simulink model "proba1"  (R2017b)
settings: Solver=VariableStepAuto  StartTime=0.0  StopTime=120  RelTol=1e-3  EnableMultiTasking=on
libraries: xbsIndex_r4 x61
settings Model: Creator=szekelyi  LastModifiedBy=kovacs.attila
settings DataIOCC: LimitDataPoints=on
settings OptimizationCC: LifeSpan=inf
settings DebuggingCC: AllowSymbolicDim=off  SFUnexpectedBacktrackingDiag=warning  SFNoUnconditionalDefaultTransitionDiag=warning  SFExecutionAtInitializationDiag=none
settings ModelReferenceCC: PropagateSignalLabelsOutOfModel=off
settings CodeAppCC: StateflowObjectComments=on
settings GRTTargetCC: TargetLangStandard=C89/C90 (ANSI)
settings ConfigComp: CovMetricSettings=dw  CovHtmlReporting=on  CovSaveCumulativeToWorkspaceVar=on  CovSaveSingleToWorkspaceVar=on  CovExternalEMLEnable=off

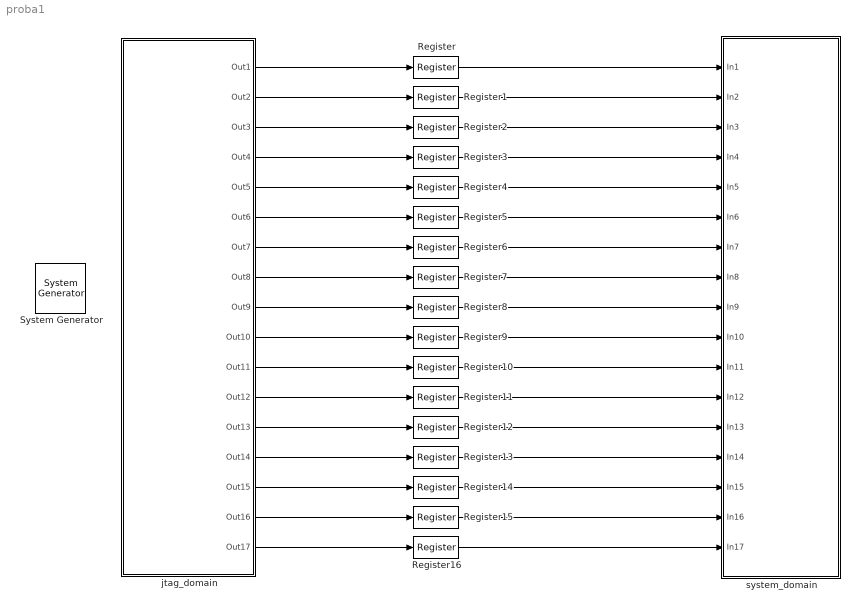
== system proba1 ==
  " System Generator" : xbsIndex_r4/ System Generator  Tag=genX  xilinxfamily=artix7  part=xc7a35t  speed=-1  package=cpg236  synthesis_tool=Vivado  clock_wrapper=Clock Enables  directory=./netlist  proj_type=Vivado  Synth_file=Vivado Synthesis Defaults  Impl_file=Vivado Implementation Defaults  testbench=off  simulink_period=1  sysclk_period=10  dcm_input_clock_period=10  incr_netlist=off  trim_vbits=Everywhere in SubSystem  dbl_ovrd=According to Block Masks  core_generation=According to Block Masks  run_coregen=off  deprecated_control=off  eval_field=0  block_type=sysgen
  Register{,1..16} (17 alike) : xbsIndex_r4/Register  init=0  rst=off  en=off  dbl_ovrd=off  block_type=register
  jtag_domain : Subsystem
  system_domain : Subsystem
  wires:
  jtag_domain/1(Out1) -> Register/1
  jtag_domain/2(Out2) -> Register1/1
  jtag_domain/3(Out3) -> Register2/1
  jtag_domain/4(Out4) -> Register3/1
  jtag_domain/5(Out5) -> Register4/1
  jtag_domain/6(Out6) -> Register5/1
  Register/1 -> system_domain/1(In1)
  Register1/1 -> system_domain/2(In2)
  Register2/1 -> system_domain/3(In3)
  Register3/1 -> system_domain/4(In4)
  Register4/1 -> system_domain/5(In5)
  Register5/1 -> system_domain/6(In6)
  Register11/1 -> system_domain/12(In12)
  Register9/1 -> system_domain/10(In10)
  jtag_domain/11(Out11) -> Register10/1
  Register10/1 -> system_domain/11(In11)
  Register8/1 -> system_domain/9(In9)
  Register7/1 -> system_domain/8(In8)
  Register6/1 -> system_domain/7(In7)
  jtag_domain/12(Out12) -> Register11/1
  jtag_domain/10(Out10) -> Register9/1
  jtag_domain/8(Out8) -> Register7/1
  jtag_domain/9(Out9) -> Register8/1
  jtag_domain/7(Out7) -> Register6/1
  Register15/1 -> system_domain/16(In16)
  jtag_domain/17(Out17) -> Register16/1
  Register16/1 -> system_domain/17(In17)
  Register14/1 -> system_domain/15(In15)
  Register13/1 -> system_domain/14(In14)
  Register12/1 -> system_domain/13(In13)
  jtag_domain/16(Out16) -> Register15/1
  jtag_domain/14(Out14) -> Register13/1
  jtag_domain/15(Out15) -> Register14/1
  jtag_domain/13(Out13) -> Register12/1

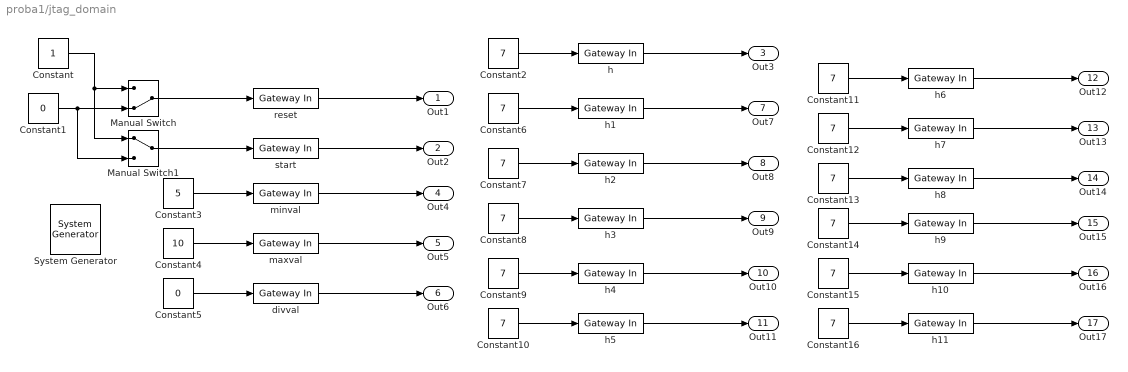
== system proba1/jtag_domain ==
  " System Generator" : xbsIndex_r4/ System Generator  Tag=genX  xilinxfamily=artix7  part=xc7a35t  speed=-1  package=cpg236  synthesis_tool=Vivado  clock_wrapper=Clock Enables  directory=./netlist  proj_type=Vivado  Synth_file=Vivado Synthesis Defaults  Impl_file=Vivado Implementation Defaults  testbench=off  simulink_period=1  sysclk_period=10  dcm_input_clock_period=10  incr_netlist=off  trim_vbits=Everywhere in SubSystem  dbl_ovrd=According to Block Masks  core_generation=According to Block Masks  run_coregen=off  deprecated_control=off  eval_field=0  block_type=sysgen
  Constant : Constant
  Constant1 : Constant  Value=0
  Constant{2,6..16} (12 alike) : Constant  Value=7
  Constant3 : Constant  Value=5
  Constant4 : Constant  Value=10
  Constant5 : Constant  Value=0
  Manual Switch : ManualSwitch  CurrentSetting=0
  Manual Switch1 : ManualSwitch
  divval : xbsIndex_r4/Gateway In  gui_display_data_type=Fixed-point  arith_type=Unsigned  n_bits=10  bin_pt=0  preci_type=Single  exp_width=8  frac_width=24  rows=1  columns=1  quantization="Round  (unbiased: +/- Inf)"  overflow=Saturate  period=1  UseAsADC=off  ADCChannel='1'  interface=None  automatic_assignment=on  address_offset=hex2dec('00')  intf_name=''  intf_description=''  default_value=0  timing_constraint=None  locs_specified=off  LOCs={}  io_standard={}  inherit_from_input=off  hdl_port=on  dbl_ovrd=off  block_type=gatewayin
  h{,1..11} (12 alike) : xbsIndex_r4/Gateway In  gui_display_data_type=Fixed-point  arith_type=Unsigned  n_bits=32  bin_pt=0  preci_type=Single  exp_width=8  frac_width=24  rows=1  columns=1  quantization="Round  (unbiased: +/- Inf)"  overflow=Saturate  period=1  UseAsADC=off  ADCChannel='1'  interface=None  automatic_assignment=on  address_offset=hex2dec('00')  intf_name=''  intf_description=''  default_value=0  timing_constraint=None  locs_specified=off  LOCs={}  io_standard={}  inherit_from_input=off  hdl_port=on  dbl_ovrd=off  block_type=gatewayin
  maxval : xbsIndex_r4/Gateway In  gui_display_data_type=Fixed-point  arith_type=Unsigned  n_bits=32  bin_pt=0  preci_type=Single  exp_width=8  frac_width=24  rows=1  columns=1  quantization="Round  (unbiased: +/- Inf)"  overflow=Saturate  period=1  UseAsADC=off  ADCChannel='1'  interface=None  automatic_assignment=on  address_offset=hex2dec('00')  intf_name=''  intf_description=''  default_value=0  timing_constraint=None  locs_specified=off  LOCs={}  io_standard={}  inherit_from_input=off  hdl_port=on  dbl_ovrd=off  block_type=gatewayin
  minval : xbsIndex_r4/Gateway In  gui_display_data_type=Fixed-point  arith_type=Unsigned  n_bits=32  bin_pt=0  preci_type=Single  exp_width=8  frac_width=24  rows=1  columns=1  quantization="Round  (unbiased: +/- Inf)"  overflow=Saturate  period=1  UseAsADC=off  ADCChannel='1'  interface=None  automatic_assignment=on  address_offset=hex2dec('00')  intf_name=''  intf_description=''  default_value=0  timing_constraint=None  locs_specified=off  LOCs={}  io_standard={}  inherit_from_input=off  hdl_port=on  dbl_ovrd=off  block_type=gatewayin
  reset : xbsIndex_r4/Gateway In  gui_display_data_type=Boolean  arith_type=Boolean  n_bits=16  bin_pt=14  preci_type=Single  exp_width=8  frac_width=24  rows=1  columns=1  quantization="Round  (unbiased: +/- Inf)"  overflow=Saturate  period=1  UseAsADC=off  ADCChannel='1'  interface=None  automatic_assignment=on  address_offset=hex2dec('00')  intf_name=''  intf_description=''  default_value=0  timing_constraint=None  locs_specified=off  LOCs={}  io_standard={}  inherit_from_input=off  hdl_port=on  dbl_ovrd=off  block_type=gatewayin
  start : xbsIndex_r4/Gateway In  gui_display_data_type=Boolean  arith_type=Boolean  n_bits=16  bin_pt=14  preci_type=Single  exp_width=8  frac_width=24  rows=1  columns=1  quantization="Round  (unbiased: +/- Inf)"  overflow=Saturate  period=1  UseAsADC=off  ADCChannel='1'  interface=None  automatic_assignment=on  address_offset=hex2dec('00')  intf_name=''  intf_description=''  default_value=0  timing_constraint=None  locs_specified=off  LOCs={}  io_standard={}  inherit_from_input=off  hdl_port=on  dbl_ovrd=off  block_type=gatewayin
  Out1 : Outport
  Out2 : Outport  Port=2
  Out3 : Outport  Port=3
  Out4 : Outport  Port=4
  Out5 : Outport  Port=5
  Out6 : Outport  Port=6
  Out7 : Outport  Port=7
  Out8 : Outport  Port=8
  Out9 : Outport  Port=9
  Out10 : Outport  Port=10
  Out11 : Outport  Port=11
  Out12 : Outport  Port=12
  Out13 : Outport  Port=13
  Out14 : Outport  Port=14
  Out15 : Outport  Port=15
  Out16 : Outport  Port=16
  Out17 : Outport  Port=17
  wires:
  h/1 -> Out3/1
  start/1 -> Out2/1
  maxval/1 -> Out5/1
  minval/1 -> Out4/1
  divval/1 -> Out6/1
  reset/1 -> Out1/1
  Manual Switch/1 -> reset/1
  Manual Switch1/1 -> start/1
  Constant/1 -> Manual Switch1/1, Manual Switch/1
  Constant1/1 -> Manual Switch1/2, Manual Switch/2
  Constant2/1 -> h/1
  Constant3/1 -> minval/1
  Constant4/1 -> maxval/1
  Constant5/1 -> divval/1
  Constant6/1 -> h1/1
  h1/1 -> Out7/1
  Constant7/1 -> h2/1
  h2/1 -> Out8/1
  Constant8/1 -> h3/1
  h3/1 -> Out9/1
  Constant9/1 -> h4/1
  h4/1 -> Out10/1
  Constant10/1 -> h5/1
  h5/1 -> Out11/1
  Constant11/1 -> h6/1
  h6/1 -> Out12/1
  Constant12/1 -> h7/1
  h7/1 -> Out13/1
  Constant13/1 -> h8/1
  h8/1 -> Out14/1
  Constant14/1 -> h9/1
  h9/1 -> Out15/1
  Constant15/1 -> h10/1
  h10/1 -> Out16/1
  Constant16/1 -> h11/1
  h11/1 -> Out17/1

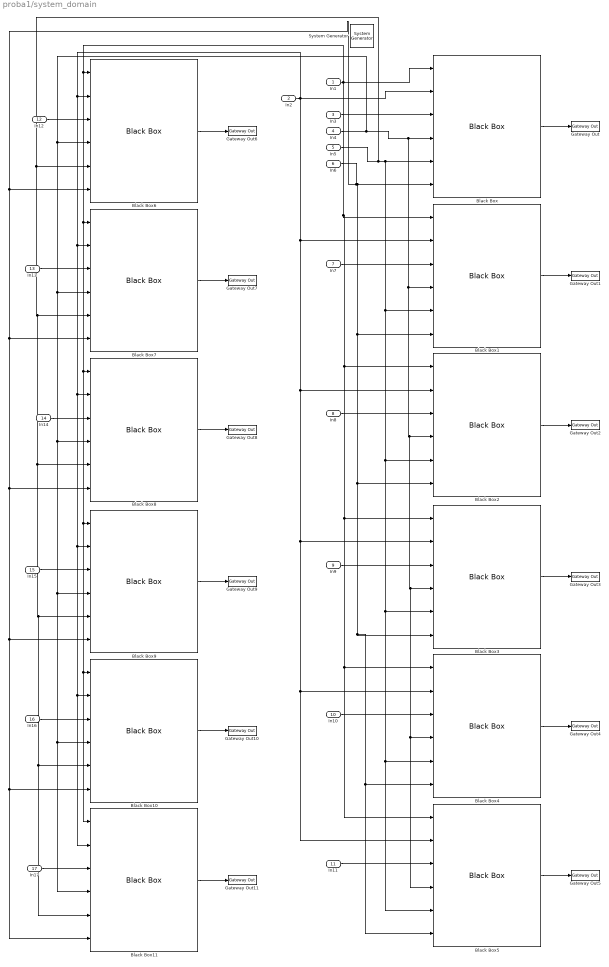
== system proba1/system_domain ==
  In1 : Inport
  In2 : Inport  Port=2
  In3 : Inport  Port=3
  In4 : Inport  Port=4
  In5 : Inport  Port=5
  In6 : Inport  Port=6
  In7 : Inport  Port=7
  In8 : Inport  Port=8
  In9 : Inport  Port=9
  In10 : Inport  Port=10
  In11 : Inport  Port=11
  In12 : Inport  Port=12
  In13 : Inport  Port=13
  In14 : Inport  Port=14
  In15 : Inport  Port=15
  In16 : Inport  Port=16
  In17 : Inport  Port=17
  " System Generator" : xbsIndex_r4/ System Generator  Tag=genX  xilinxfamily=artix7  part=xc7a35t  speed=-1  package=cpg236  synthesis_tool=Vivado  clock_wrapper=Clock Enables  directory=./netlist  proj_type=Vivado  Synth_file=Vivado Synthesis Defaults  Impl_file=Vivado Implementation Defaults  testbench=off  simulink_period=1  sysclk_period=10  dcm_input_clock_period=10  incr_netlist=off  trim_vbits=Everywhere in SubSystem  dbl_ovrd=According to Block Masks  core_generation=According to Block Masks  run_coregen=off  deprecated_control=off  eval_field=0  block_type=sysgen
  Black Box{,1..11} (12 alike) : xbsIndex_r4/Black Box  init_code=pwm_ultra_config  sim_method=ISE Simulator  verbose=off  block_type=blackbox2
  Gateway Out : xbsIndex_r4/Gateway Out  inherit_from_input=off  hdl_port=on  rows=1  columns=1  UseAsDAC=off  DACChannel='1'  interface=None  automatic_assignment=on  address_offset=hex2dec('00')  intf_name=''  intf_description=''  timing_constraint=None  locs_specified=on  LOCs={'M3'}  io_standard={'LVCMOS33'}  block_type=gatewayout
  Gateway Out1 : xbsIndex_r4/Gateway Out  inherit_from_input=off  hdl_port=on  rows=1  columns=1  UseAsDAC=off  DACChannel='1'  interface=None  automatic_assignment=on  address_offset=hex2dec('00')  intf_name=''  intf_description=''  timing_constraint=None  locs_specified=on  LOCs={'L3'}  io_standard={'LVCMOS33'}  block_type=gatewayout
  Gateway Out10 : xbsIndex_r4/Gateway Out  inherit_from_input=off  hdl_port=on  rows=1  columns=1  UseAsDAC=off  DACChannel='1'  interface=None  automatic_assignment=on  address_offset=hex2dec('00')  intf_name=''  intf_description=''  timing_constraint=None  locs_specified=on  LOCs={'J1'}  io_standard={'LVCMOS33'}  block_type=gatewayout
  Gateway Out11 : xbsIndex_r4/Gateway Out  inherit_from_input=off  hdl_port=on  rows=1  columns=1  UseAsDAC=off  DACChannel='1'  interface=None  automatic_assignment=on  address_offset=hex2dec('00')  intf_name=''  intf_description=''  timing_constraint=None  locs_specified=on  LOCs={'K2'}  io_standard={'LVCMOS33'}  block_type=gatewayout
  Gateway Out2 : xbsIndex_r4/Gateway Out  inherit_from_input=off  hdl_port=on  rows=1  columns=1  UseAsDAC=off  DACChannel='1'  interface=None  automatic_assignment=on  address_offset=hex2dec('00')  intf_name=''  intf_description=''  timing_constraint=None  locs_specified=on  LOCs={'A16'}  io_standard={'LVCMOS33'}  block_type=gatewayout
  Gateway Out3 : xbsIndex_r4/Gateway Out  inherit_from_input=off  hdl_port=on  rows=1  columns=1  UseAsDAC=off  DACChannel='1'  interface=None  automatic_assignment=on  address_offset=hex2dec('00')  intf_name=''  intf_description=''  timing_constraint=None  locs_specified=on  LOCs={'K3'}  io_standard={'LVCMOS33'}  block_type=gatewayout
  Gateway Out4 : xbsIndex_r4/Gateway Out  inherit_from_input=off  hdl_port=on  rows=1  columns=1  UseAsDAC=off  DACChannel='1'  interface=None  automatic_assignment=on  address_offset=hex2dec('00')  intf_name=''  intf_description=''  timing_constraint=None  locs_specified=on  LOCs={'C15'}  io_standard={'LVCMOS33'}  block_type=gatewayout
  Gateway Out5 : xbsIndex_r4/Gateway Out  inherit_from_input=off  hdl_port=on  rows=1  columns=1  UseAsDAC=off  DACChannel='1'  interface=None  automatic_assignment=on  address_offset=hex2dec('00')  intf_name=''  intf_description=''  timing_constraint=None  locs_specified=on  LOCs={'H1'}  io_standard={'LVCMOS33'}  block_type=gatewayout
  Gateway Out6 : xbsIndex_r4/Gateway Out  inherit_from_input=off  hdl_port=on  rows=1  columns=1  UseAsDAC=off  DACChannel='1'  interface=None  automatic_assignment=on  address_offset=hex2dec('00')  intf_name=''  intf_description=''  timing_constraint=None  locs_specified=on  LOCs={'A15'}  io_standard={'LVCMOS33'}  block_type=gatewayout
  Gateway Out7 : xbsIndex_r4/Gateway Out  inherit_from_input=off  hdl_port=on  rows=1  columns=1  UseAsDAC=off  DACChannel='1'  interface=None  automatic_assignment=on  address_offset=hex2dec('00')  intf_name=''  intf_description=''  timing_constraint=None  locs_specified=on  LOCs={'B15'}  io_standard={'LVCMOS33'}  block_type=gatewayout
  Gateway Out8 : xbsIndex_r4/Gateway Out  inherit_from_input=off  hdl_port=on  rows=1  columns=1  UseAsDAC=off  DACChannel='1'  interface=None  automatic_assignment=on  address_offset=hex2dec('00')  intf_name=''  intf_description=''  timing_constraint=None  locs_specified=on  LOCs={'A14'}  io_standard={'LVCMOS33'}  block_type=gatewayout
  Gateway Out9 : xbsIndex_r4/Gateway Out  inherit_from_input=off  hdl_port=on  rows=1  columns=1  UseAsDAC=off  DACChannel='1'  interface=None  automatic_assignment=on  address_offset=hex2dec('00')  intf_name=''  intf_description=''  timing_constraint=None  locs_specified=on  LOCs={'J3'}  io_standard={'LVCMOS33'}  block_type=gatewayout
  wires:
  Black Box/1 -> Gateway Out/1
  In4/1 -> Black Box11/4, Black Box10/4, Black Box9/4, Black Box8/4, Black Box7/4, Black Box6/4, Black Box5/4, Black Box4/4, Black Box3/4, Black Box2/4, Black Box1/4, Black Box/4
  In2/1 -> Black Box5/2, Black Box4/2, Black Box3/2, Black Box2/2, Black Box1/2, Black Box11/2, Black Box10/2, Black Box9/2, Black Box8/2, Black Box7/2, Black Box6/2, Black Box/2
  In6/1 -> Black Box5/6, Black Box4/6, Black Box3/6, Black Box2/6, Black Box1/6, Black Box/6, Black Box11/6, Black Box10/6, Black Box9/6, Black Box8/6, Black Box7/6, Black Box6/6
  In5/1 -> Black Box11/5, Black Box10/5, Black Box9/5, Black Box8/5, Black Box7/5, Black Box6/5, Black Box5/5, Black Box4/5, Black Box3/5, Black Box2/5, Black Box1/5, Black Box/5
  In3/1 -> Black Box/3
  In1/1 -> Black Box5/1, Black Box4/1, Black Box3/1, Black Box2/1, Black Box1/1, Black Box11/1, Black Box10/1, Black Box9/1, Black Box8/1, Black Box7/1, Black Box6/1, Black Box/1
  Black Box1/1 -> Gateway Out1/1
  Black Box2/1 -> Gateway Out2/1
  Black Box3/1 -> Gateway Out3/1
  Black Box4/1 -> Gateway Out4/1
  Black Box5/1 -> Gateway Out5/1
  Black Box6/1 -> Gateway Out6/1
  Black Box10/1 -> Gateway Out10/1
  Black Box8/1 -> Gateway Out8/1
  Black Box7/1 -> Gateway Out7/1
  Black Box9/1 -> Gateway Out9/1
  Black Box11/1 -> Gateway Out11/1
  In7/1 -> Black Box1/3
  In8/1 -> Black Box2/3
  In9/1 -> Black Box3/3
  In10/1 -> Black Box4/3
  In11/1 -> Black Box5/3
  In12/1 -> Black Box6/3
  In13/1 -> Black Box7/3
  In14/1 -> Black Box8/3
  In15/1 -> Black Box9/3
  In16/1 -> Black Box10/3
  In17/1 -> Black Box11/3
